simulink model "lek9"  (Simulink 7.5)
settings: Solver=ode45  StartTime=0.0  StopTime=10.0  RelTol=1e-3
values from neighbouring files (symbols this model uses):
  A = [-1 -3 0; 0 1 1; 0 2 0]    [Lektion9.m]    (also in lek8.m = [-1.5 0.2; 0.13 0])
  B = [1 2/3; 0 1/3; 0 1/3]    [Lektion9.m]    (also in lek8.m = [1 0; 1 -1])
  K = 4.47*10^-4    (= 0.000447)    [portefoelje.m]
undefined symbols (not defined in the file or in its folder): C, L, xd
libraries: simulink x1
settings Model: Creator=Aq  LastModifiedBy=Aq

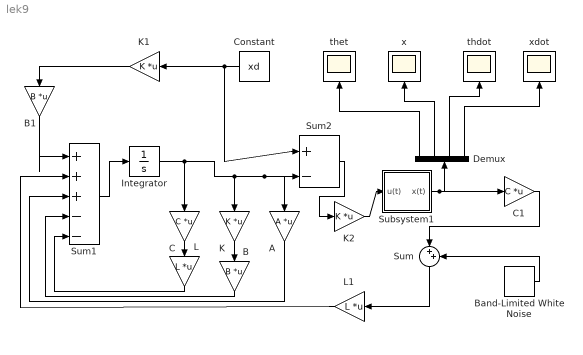
== system lek9 ==
  A : Gain  Gain=A  Multiplication=Matrix(K*u)  ParameterDataType=fixdt(1, 16)  ParameterScaling=2^0  OutDataType=fixdt(1, 16)  OutScaling=2^0
  B : Gain  Gain=B  Multiplication=Matrix(K*u)  ParameterDataType=fixdt(1, 16)  ParameterScaling=2^0  OutDataType=fixdt(1, 16)  OutScaling=2^0
  B1 : Gain  Gain=B  Multiplication=Matrix(K*u)  ParameterDataType=fixdt(1, 16)  ParameterScaling=2^0  OutDataType=fixdt(1, 16)  OutScaling=2^0
  Band-Limited White Noise : simulink/Sources/Band-Limited White Noise  SystemSampleTime=-1  Cov=[0.000000001]  Ts=0.1  seed=[23341]
  C : Gain  Gain=C  Multiplication=Matrix(K*u)  ParameterDataType=fixdt(1, 16)  ParameterScaling=2^0  OutDataType=fixdt(1, 16)  OutScaling=2^0
  C1 : Gain  Gain=C  Multiplication=Matrix(K*u)  ParameterDataType=fixdt(1, 16)  ParameterScaling=2^0  OutDataType=fixdt(1, 16)  OutScaling=2^0
  Constant : Constant  Value=xd  OutDataType=fixdt(1, 16)  OutScaling=2^0
  Demux : Demux
  Integrator : Integrator
  K : Gain  Gain=K  Multiplication=Matrix(K*u)  ParameterDataType=fixdt(1, 16)  ParameterScaling=2^0  OutDataType=fixdt(1, 16)  OutScaling=2^0
  K1 : Gain  Gain=K  Multiplication=Matrix(K*u)  ParameterDataType=fixdt(1, 16)  ParameterScaling=2^0  OutDataType=fixdt(1, 16)  OutScaling=2^0
  K2 : Gain  Gain=K  Multiplication=Matrix(K*u)  ParameterDataType=fixdt(1, 16)  ParameterScaling=2^0  OutDataType=fixdt(1, 16)  OutScaling=2^0
  L : Gain  Gain=L  Multiplication=Matrix(K*u)  ParameterDataType=fixdt(1, 16)  ParameterScaling=2^0  OutDataType=fixdt(1, 16)  OutScaling=2^0
  L1 : Gain  Gain=L  Multiplication=Matrix(K*u)  ParameterDataType=fixdt(1, 16)  ParameterScaling=2^0  OutDataType=fixdt(1, 16)  OutScaling=2^0
  Subsystem1 : Subsystem
  Sum : Sum  Inputs=|++  OutDataType=fixdt(1, 16)  OutScaling=2^0
  Sum1 : Sum  Inputs=|+++--  OutDataType=fixdt(1, 16)  OutScaling=2^0
  Sum2 : Sum  Inputs=|+-  OutDataType=fixdt(1, 16)  OutScaling=2^0
  thdot : Scope
      settings: SaveName=ScopeData2
  thet : Scope
  x : Scope
  xdot : Scope
      settings: SaveName=ScopeData3
  wires:
  Demux/4 -> xdot/1
  Demux/2 -> x/1
  Demux/1 -> thet/1
  Demux/3 -> thdot/1
  Subsystem1/1(x(t)) -> C1/1, Demux/1
  C1/1 -> Sum/1
  Sum/1 -> L1/1
  L1/1 -> Sum1/2
  L/1 -> Sum1/5
  B/1 -> Sum1/4
  A/1 -> Sum1/3
  B1/1 -> Sum1/1
  K1/1 -> B1/1
  Constant/1 -> K1/1, Sum2/1
  Integrator/1 -> C/1, Sum2/2, A/1, K/1
  K/1 -> B/1
  C/1 -> L/1
  Sum1/1 -> Integrator/1
  Sum2/1 -> K2/1
  K2/1 -> Subsystem1/1(u(t))
  Band-Limited White Noise/1 -> Sum/2

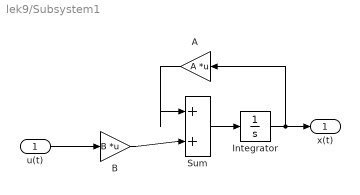
== system lek9/Subsystem1 ==
  u(t) : Inport  OutDataType=fixdt(1, 16)  OutScaling=2^0
  A : Gain  Gain=A  Multiplication=Matrix(K*u)  ParameterDataType=fixdt(1, 16)  ParameterScaling=2^0  OutDataType=fixdt(1, 16)  OutScaling=2^0
  B : Gain  Gain=B  Multiplication=Matrix(K*u)  ParameterDataType=fixdt(1, 16)  ParameterScaling=2^0  OutDataType=fixdt(1, 16)  OutScaling=2^0
  Integrator : Integrator
  Sum : Sum  Inputs=|++  OutDataType=fixdt(1, 16)  OutScaling=2^0
  x(t) : Outport  OutDataType=fixdt(1, 16)  OutScaling=2^0
  wires:
  A/1 -> Sum/1
  Integrator/1 -> x(t)/1, A/1
  Sum/1 -> Integrator/1
  B/1 -> Sum/2
  u(t)/1 -> B/1
